simulink library "SpeedBumpLibrary"  (R2023b)
settings: Solver=VariableStepAuto  StartTime=0.0  StopTime=10.0  RelTol=1e-3
values from neighbouring files (symbols this model uses):
  a = 1.35    [Parameters.m]
  b = 1.5    [Parameters.m]
settings Model: Creator=arturogonzalez  LastModifiedBy=franc
settings SolverCC: AlgebraicLoopSolver=TrustRegion
settings DebuggingCC: UnconnectedInputMsg=warning  UnconnectedOutputMsg=warning  UnconnectedLineMsg=warning
settings ModelReferenceCC: EnableRefExpFcnMdlSchedulingChecks=on

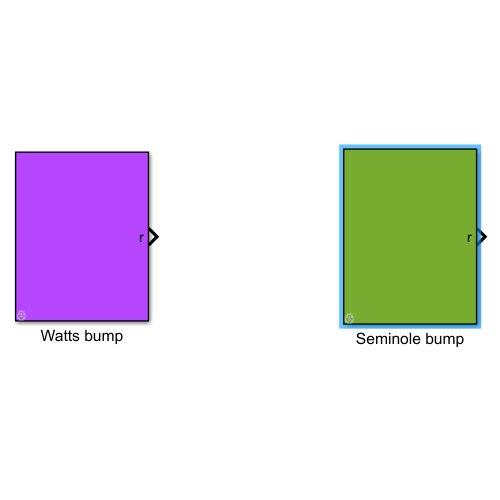
[thumbnail: Simulink's stored preview of the top-level diagram]
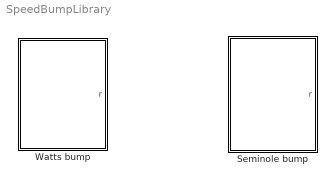
== system SpeedBumpLibrary ==
  Seminole bump : Subsystem  mask{h=0.1, d=3, L=6.7, v=8, delta=a+b, n=5}
      mask prompts: h "Bump height (m)"; d "Top length (m)"; L "Bump length (m)"; v "Vehicle speed (m/s)"; delta "Inter axis (m)"; n "Bump number"
  Watts bump : Subsystem  mask{h=0.1, L=3.7, v=8, delta=0, n=10}
      mask prompts: h "Bump height (m)"; L "Bump length (m)"; v "Vehicle speed (m/s)"; delta "Inter axis (m)"; n "Bump number"

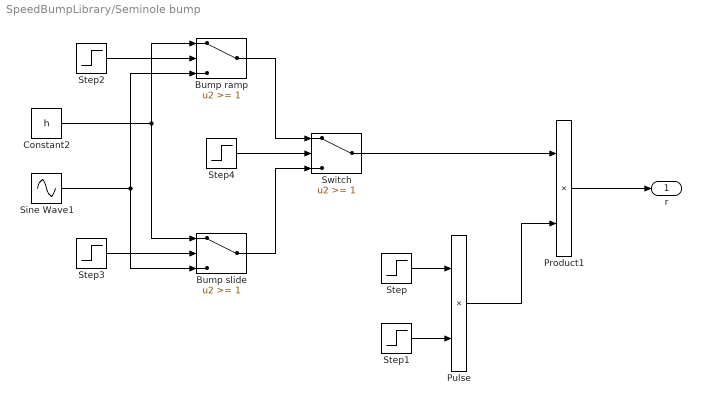
== system SpeedBumpLibrary/Seminole bump ==
  Bump ramp : Switch  Threshold=1  SaturateOnIntegerOverflow=off  InputSameDT=off
  Bump slide : Switch  Threshold=1  SaturateOnIntegerOverflow=off  InputSameDT=off
  Constant2 : Constant  Value=h
  Product1 : Product
  Pulse : Product
  Sine Wave1 : Sin  Amplitude=h  Frequency=2*pi*(v/L)  Phase=-2*pi*(delta/L)  SampleTime=0
  Step : Step  Time=n*(L/v)+(delta/v)  SampleTime=0
  Step1 : Step  Time=(n+d+0.5)*(L/v)+(delta/v)  Before=1  After=0  SampleTime=0
  Step2 : Step  Time=(n+0.25)*(L/v)+(delta/v)  SampleTime=0
  Step3 : Step  Time=(n+d+0.25)*(L/v)+(delta/v)  Before=1  After=0  SampleTime=0
  Step4 : Step  Time=(n+d/2+0.25)*(L/v)+(delta/v)  Before=1  After=0  SampleTime=0
  Switch : Switch  Threshold=1  SaturateOnIntegerOverflow=off  InputSameDT=off
  r : Outport
  wires:
  Step4/1 -> Switch/2
  Bump slide/1 -> Switch/3
  Step3/1 -> Bump slide/2
  Bump ramp/1 -> Switch/1
  Constant2/1 -> Bump ramp/1, Bump slide/1
  Step2/1 -> Bump ramp/2
  Switch/1 -> Product1/1
  Sine Wave1/1 -> Bump ramp/3, Bump slide/3
  Step/1 -> Pulse/1
  Step1/1 -> Pulse/2
  Product1/1 -> r/1
  Pulse/1 -> Product1/2

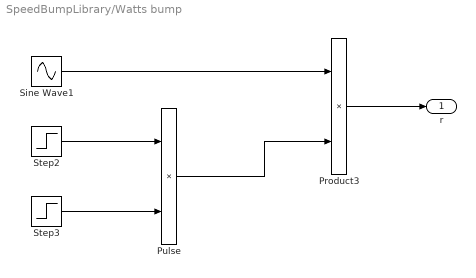
== system SpeedBumpLibrary/Watts bump ==
  Product3 : Product
  Pulse : Product
  Sine Wave1 : Sin  Amplitude=h  Frequency=2*pi*(v/L)  Phase=-2*pi*(delta/L)  SampleTime=0
  Step2 : Step  Time=n*(L/v)+(delta/v)  SampleTime=0
  Step3 : Step  Time=(n+0.5)*(L/v)+(delta/v)  Before=1  After=0  SampleTime=0
  r : Outport
  wires:
  Product3/1 -> r/1
  Pulse/1 -> Product3/2
  Step2/1 -> Pulse/1
  Step3/1 -> Pulse/2
  Sine Wave1/1 -> Product3/1
